simulink model "LQR_imple"  (R2024b)
settings: Solver=VariableStepAuto  StartTime=0.0  StopTime=T_final  RelTol=1e-3
values from neighbouring files (symbols this model uses):
  Ap = [ ... (first row only)    [lqr_implement.m]
  Ar = [ ... (first row only)    [lqr_implement.m]
  Bp = [0; 0; b_p3; b_p4; 1]    [lqr_implement.m]
  Br = [0; 0; b_r3; b_r4; 1]    [lqr_implement.m]
  ic_p = [20 ... (first row only)    [lqr_implement.m]
  ic_r = [10 ... (first row only)    [lqr_implement.m]
undefined symbols (not defined in the file or in its folder): Kp, Kr
settings Model: Creator=Ruchi  LastModifiedBy=yugan

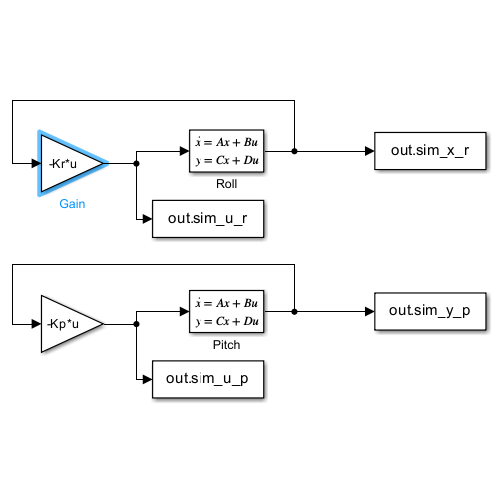
[thumbnail: Simulink's stored preview of the top-level diagram]
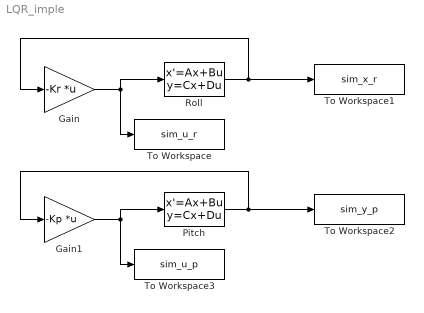
== system LQR_imple ==
  Gain : Gain  Gain=-Kr  Multiplication=Matrix(K*u)
  Gain1 : Gain  Gain=-Kp  Multiplication=Matrix(K*u)
  Pitch : StateSpace  A=Ap  B=Bp  C=eye(5)  D=zeros(5,1)  InitialCondition=ic_p
  Roll : StateSpace  A=Ar  B=Br  C=eye(5)  D=zeros(5,1)  InitialCondition=ic_r
  To Workspace : ToWorkspace  VariableName=sim_u_r  SampleTime=-1
  To Workspace1 : ToWorkspace  VariableName=sim_x_r  SampleTime=-1
  To Workspace2 : ToWorkspace  VariableName=sim_y_p  SampleTime=-1
  To Workspace3 : ToWorkspace  VariableName=sim_u_p  SampleTime=-1
  wires:
  Gain/1 -> Roll/1, To Workspace/1
  Gain1/1 -> Pitch/1, To Workspace3/1
  Roll/1 -> To Workspace1/1, Gain/1
  Pitch/1 -> To Workspace2/1, Gain1/1
